simulink library "GOcontroll_Moduline_Target"  (R2018b)
settings: Solver=ode45  StartTime=0.0  StopTime=10.0  RelTol=1e-3  EnableMultiTasking=on
(part 1 of 3)
settings Model: Creator=HANcoder  LastModifiedBy=maud
settings Model: ModifiedHistory=|
  | la_obwlf -- Thu Sep 01 12:12:55 2016 -- Version 0.33
  | 
  | 
  | 
  | 
  | 
  | 
  | la_obwlf -- Thu Sep 01 09:23:34 2016 -- Version 0.33
  | changed the version in the Base Sample Time block
  | 
  | 
  | 
  | la_obwlf -- Tue Aug 30 15:48:17 2016 -- Version 0.33
settings DataIOCC: LimitDataPoints=on  SaveFormat=Array  SignalLoggingSaveFormat=ModelDataLogs
settings OptimizationCC: ExpressionDepthLimit=2147483647  LifeSpan=inf
settings DebuggingCC: UnderspecifiedInitializationDetection=Classic  MergeDetectMultiDrivingBlocksExec=none  SolverPrmCheckMsg=warning  FcnCallInpInsideContextMsg=warning  StateNameClashWarn=warning  SFUnexpectedBacktrackingDiag=warning  SFNoUnconditionalDefaultTransitionDiag=warning  SFExecutionAtInitializationDiag=none
settings HardwareCC: ProdBitPerPointer=32  ProdBitPerSizeT=32  ProdBitPerPtrDiffT=32  ProdLargestAtomicFloat=None  ProdIntDivRoundTo=Undefined  ProdEndianess=Unspecified  ProdWordSize=32  ProdHWDeviceType=32-bit Generic
settings ModelReferenceCC: PropagateSignalLabelsOutOfModel=off
settings SFSimCC: SimUseLocalCustomCode=off
settings RTWCC: RTWUseLocalCustomCode=off
settings CodeAppCC: StateflowObjectComments=on
settings GRTTargetCC: TargetLangStandard=C89/C90 (ANSI)  GeneratePreprocessorConditionals=Disable all  CombineOutputUpdateFcns=off  GRTInterface=on
settings ConfigComp: CovMetricSettings=dw  CovHtmlReporting=on  CovSaveCumulativeToWorkspaceVar=on  CovSaveSingleToWorkspaceVar=on  CovExternalEMLEnable=off  CovSFcnEnable=off

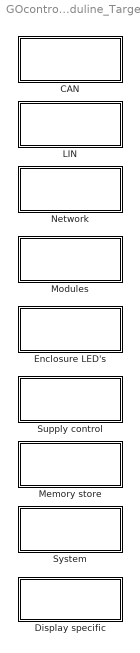
== system GOcontroll_Moduline_Target ==
  CAN : Subsystem
      mask Display: fprintf('CAN');
  Display specific : Subsystem
      mask Display: fprintf("Display specific");
  Enclosure LED's : Subsystem
      mask Display: fprintf('Enclosure LED');
  LIN : Subsystem
      mask Display: fprintf('LIN');
  Memory store : Subsystem
      mask Display: fprintf('Memory store');
  Modules : Subsystem
      mask Display: fprintf('Modules');
  Network : Subsystem
      mask Display: fprintf('Network');
  Supply control : Subsystem
      mask Display: fprintf('Supply Control');
  System : Subsystem
      mask Display: fprintf('System');

== system GOcontroll_Moduline_Target/CAN ==
  CAN 2.0B : Subsystem
      mask Display: fprintf('CAN 2.0B');

== system GOcontroll_Moduline_Target/Display specific ==
  Set display brightness : Subsystem  mask{tsamp=0}
      mask prompts: tsamp "Sample time:"
      mask help:
      | Set the brightness of a display (only works with the max25014 driver currently)
      | Keeps the original brightness untill the first non zero value is received
      mask init:
      | sfcn_set_brightness_display_mcb();
      mask Display:
      | fprintf("Set display brightness");
      | text(2, 6, ert_linux_target_version());

== system GOcontroll_Moduline_Target/Enclosure LED's ==
  Enclosure LED : Subsystem  Tag=HANcoder_GOcontroll_Moduline_IV  mask(Enclosure LED's){led=1, color=Red}
      mask help:
      | The Moduline controller is equipped with 4 RGB status LED's. To control them, simply configure the mask ( LED and color) and control them using uint8 values.
      |
      | Note: Moduline IV HW >= 3.02 has duty cycle controlled LED's. The intensity can be set from 0 (0%) to 255 (100%).
      |
      | LED: Select the LED that is needs to be controlled.
      |
      | Color: Select the color the LED needs to illuminate.
      mask init:
      | [colorInfoStr] = sfcn_gocontroll_status_led_mcb(led, color);
      mask TypeOptions led: 1 | 2 | 3 | 4
      mask TypeOptions color: Red | Green | Blue
      mask Display:
      | fprintf('Status LED %d\nColor: %s',led,colorInfoStr);
      | text(2, 6, ert_linux_target_version());

== system GOcontroll_Moduline_Target/LIN ==
  LIN Master : Subsystem  Tag=HANcoder_GOcontroll_Moduline_IV  mask(LIN Master){id=0x01, direction=Send data, dataLength=4, check=Classic (LIN 1.3), tsamp=-1}
      mask prompts: id "Identifier"; dataLength "Data Length"; check "Checksum"; tsamp "Sample time"
      mask help:
      | Function
      | ==========
      | This block implements the LIN master functionality for communication with LIN
      | slaves. The block complies with LIN 1.3 an LIN 2.0. When sending data to a slave
      | device, this block will add the data to the LIN bus. When retrieving data from slaves, The block will wait for incoming data over LIN.
      |
      | Parameters
      | ==========
      | Identifier:
      | Selects the identifier to communicate with
      |
      | Direction:
      | Request data from a slave device or send data to a slave device
      |
      | Datalength:
      | Defines the number of bytes that need to be send to- or requested from the slave
      |
      | Checksum:
      | Select Classic for checksum based on databytes only. Enhanced for databytes and
      | ID byte
      |
      | Sample time:
      | Defines the execution interval of the block.
      |
      | Input
      | ==========
      | Port 1..8               LIN Data bytes to be send to a slave
      |
      | Output
      | ==========
      | Port 1..8               LIN Data bytes that are received from the slave
      mask init:
      | sfcn_lin_master_mcb(id, direction, dataLength, check)
      mask TypeOptions id: 0x01 | 0x02 | 0x03 | 0x04 | 0x05 | 0x06 | 0x07 | 0x08 | 0x09 | 0x0A | 0x0B | 0x0C | 0x0D | 0x0E | 0x0F | 0x10 | 0x11 | 0x12 | 0x13 | 0x14 | 0x15 | 0x16 | 0x17 | 0x18 | 0x19 | 0x1A | 0x1B | 0x1C | 0x1D | 0x1E | 0x1F | 0x20 | 0x21 | 0x22 | 0x23 | 0x24 | 0x25 | 0x26 | 0x27 | 0x28 | 0x29 | 0x2A | 0x2B | 0x2C | 0x2D | 0x2E | 0x2F | 0x30 | 0x31 | 0x32 | 0x33 | 0x34 | 0x35 | 0x36 | 0x37 | 0x38 | 0x39 | 0x3A | 0x3B | 0x3C (diagnostic) | 0x3D (diagnostic) | 0x3E (reserved) | 0x3F (reserved)
      mask TypeOptions direction: Request data | Send data
      mask TypeOptions dataLength: 2 | 4 | 8
      mask TypeOptions check: Classic (LIN 1.3) | Enhanced (LIN 2.0)
      mask Display:
      | fprintf('Master LIN\nmessage\nID: 0x%x',id);
      | text(2, 6, ert_linux_target_version());

== system GOcontroll_Moduline_Target/Memory store ==
  Diagnostic to memory : Subsystem
      mask Display: fprintf('Diagnostic to memory');
  Variable to memory : Subsystem
      mask Display: fprintf('Variable to memory');

== system GOcontroll_Moduline_Target/Modules ==
  Bridge Module : Subsystem
      mask Display: fprintf('Bridge Module');
  Input Module : Subsystem
      mask Display: fprintf('Input Module');
  Output Module : Subsystem
      mask Display: fprintf('Output Module');

== system GOcontroll_Moduline_Target/Network ==
  MQTT : Subsystem
      mask Display: fprintf('MQTT');
  UDP : Subsystem
      mask Display: fprintf('UDP');

== system GOcontroll_Moduline_Target/Supply control ==
  Controller Active : Subsystem  Tag=HANcoder_GOcontroll_Moduline_IV  mask(Controller Active){tsamp=1}
      mask prompts: tsamp "Sample time"
      mask help:
      | The GOcontroll Moduline IV is able to keep itself alive. As long the K30 power is applied (connector C pin 5-7) and the input of the Controller Active function block is high, the controller will stay on even if the K15 pins (connector C pin 2,3 or 4) are low.
      | If the controller is switched off by software, a restart is only possible when the device is activated by one of the K15 pins of connector C.
      |
      | To detect an external shutdown (K15 pins goes low), simply drag in the K15 Voltage block. This block provides the input voltage from the K15 pins
      mask init:
      | sfcn_gocontroll_controller_active_mcb();
      mask Display:
      | fprintf('Controller Active');
      | text(2, 6, ert_linux_target_version());
  K15 Voltage : Subsystem  Tag=HANcoder_GOcontroll_Moduline_IV  mask(Contact Voltage){tsamp=1, k15pin=K15-1 (Connector C pin 2)}
      mask prompts: tsamp "Sample time"; k15pin "K15 input pin"
      mask help: The K15 voltage provides the K15 voltage in mV that is applied on connector C pin 2,3 or 4. A positive voltage on one of these pins will start-up the controller. These function blocks can be used to read out which K15 input pin triggered the startup.
      mask init:
      | sfcn_gocontroll_k15_voltage_mcb(k15pin);
      mask TypeOptions k15pin: K15-1 (Connector C pin 2) | K15-2 (Connector C pin 3) | K15-3 (Connector C pin 4)
      mask Display:
      | fprintf('K15 Voltage\nConnector C pin %d',k15pin+1);
      | text(2, 6, ert_linux_target_version());
  K30 Voltage : Subsystem  Tag=HANcoder_GOcontroll_Moduline_IV  mask(Supply voltage){tsamp=1}
      mask prompts: tsamp "Sample time"
      mask help: The K30 voltage provides the power supply in mV that is applied on connector C pin 5-7
      mask init:
      | sfcn_gocontroll_k30_voltage_mcb();
      mask Display:
      | fprintf('K30 Voltage\nConnector C pin 5-7');
      | text(2, 6, ert_linux_target_version());

== system GOcontroll_Moduline_Target/System ==
  Build Settings : Subsystem  Tag=HANcoder_GOcontroll_Moduline_IV  mask{AutoASAP2add=on, AutoFlash=off}
      mask prompts: AutoASAP2add "Add signals and parameters automatically"; AutoFlash "Automatic flash after build"
      mask TypeOptions AutoASAP2add: on | off
      mask TypeOptions AutoFlash: off | USB | CAN | Ethernet
      mask DialogControl ParameterTabVar0 Prompt: Auto Add
      mask DialogControl Control3 Prompt: With this option the undefined parameters and signals will automatically be added to the workspace for use with HANtune. You will be prompted for the parameter values.
      mask DialogControl ParameterTabVar01 Prompt: Auto Flash
      mask DialogControl Control2 Prompt: With this option you can choose to automatically start MicroBoot after the build is complete. MicroBoot will start flashing using the selected interface.
      mask Display:
      | fprintf('Build settings\nAuto Add: %s\nAuto Flash: %s',AutoASAP2add, AutoFlash);
      | text(2, 6, ert_linux_target_version());
  CPU : Subsystem  Tag=HANcoder_GOcontroll_Moduline_IV  mask(Get CPU temperature){tsamp=1}
      mask prompts: tsamp "Sample time"
      mask help: Function block to retrieve the CPU temperature from the i.MX core
      mask init:
      | sfcn_gocontroll_cpu_temperature_mcb();
      mask Display:
      | fprintf('Get CPU temperature');
      | text(2, 6, ert_linux_target_version());
  Execute Shell Command : M-S-Function  FunctionName=sfcn_exec_shell  Parameters=tsamp,command  mask{command=command, tsamp=1}
      mask prompts: tsamp "Sample time:"
      mask help: Execute a Linux Shell command when the input is true
      mask init:
      | sfcn_exec_shell_mcb(command);
      mask Help: Accepts a Boolean input, potentially use a triggered subsystem to call the function only once on a state change.
      mask Display:
      | fprintf("Execute command:\n%s",command);
      | text(2, 6, ert_linux_target_version());
  License Key : Subsystem  Tag=HANcoder_GOcontroll_Moduline_IV  mask(Check software license key){tsamp=1, key=key, iv=initVec, license=/path/to/file, check_file=/path/to/file}
      mask prompts: tsamp "Sample time"; key "Encryption key"; iv "Initialisation vector"; license "License file"; check_file "Check file"
      mask help: Function block to check the controller for a license key upon executing the software.
      mask init:
      | sfcn_license_key_mcb(key,iv,license,check_file);
      mask Help:
      | example lines are literal,  {}s need to be present in the text fields.
      | 
      | Encryption key:
      | 
      | An array of 16, 24 or 32 bytes, for example:
      | {0x01, 0x23, 0x45, 0x67, 0x89, 0xAB, 0xCD, 0xEF, 0x01, 0x23, 0x45, 0x67, 0x89, 0xAB, 0xCD, 0xEF}
      | 
      | bytes can be written in any form accepted by the c compiler: 0x00/0 to 0xFf/255.
      | 
      | Inititialisation vector:
      | 
      | A string of characters (max 16 bytes) example:
      | 123kdgh34ndfg84
      | 
      | 
      | License file:
      | 
      | A string containing the path to the license file, example:
      | /etc/simulink/license
      | 
      | 
      | Check file:
      | 
      | A string containing the path to the license file, example:
      | /etc/simulink/check_file
      | 
      | 
      | Method of operation:
      | This block uses the <a href="https://github.com/jhjin/OpenAES">OpenAES library</a>. It also has a tool that can be used to generate an encryption key and to encrypt a file with said key.
      | 
      | This block will attempt to decrypt the "license file" with the given key and initialisation vector, it will then be compared to the "check file". If these match the program is allowed to continue.
      | 
      | To make this work effectively it is essential to encrypt a file that is unique for the system and can't be easily edited. for example "/sys/class/net/eth0/address".
      | 
      | An important note with using this block is that the bytes of the key are swapped and so need to be entered slightly differently in this block, for example:
      | key: byte 1 byte 2 byte 3 byte 4 byte 5 byte 6 ...
      | block: {byte 2, byte 1, byte 4, byte 3, byte 6, byte 5, ...}
      | 
      | If the model terminates with the error:
      | Error: Failed to decrypt2. return code: ##
      | 
      | It means the license key is faulty and needs to be checked in the block.
      | it might be that your system does display the key in the right order for the block, so if this error happens first double check, then try swapping them to the regular order.
      mask Display:
      | fprintf('Check software license');
      | text(2, 6, ert_linux_target_version());

== system GOcontroll_Moduline_Target/CAN/CAN 2.0B ==
  CAN receive1 : Subsystem  Tag=HANcoder_GOcontroll_Moduline_IV  mask(CAN receive){canBus=CAN1 - Connector C pin 14 (L) and pin 15 (H), outputNumber=1, dataType=uint8, byteOrder=on, tsamp=-1}
      mask prompts: canBus "CAN channel"; outputNumber "Output ports"; dataType "Output datatype"; byteOrder "Byte order: Checked = MSB first, unchecked = LSB first."; tsamp "Sample time"
      mask help:
      | Function
      | ==========
      | Receive the newest message from the specified CAN channel.
      |
      | Parameters
      | ==========
      | CAN channel:             The CAN channel to send the message on.
      | Output ports:             The amount of output ports
      | Output datatype:       The datatype of the output ports
      | Byte order:                 Select MSB or LSB first
      | Sample time:              -1 or divisible by base sample time [seconds]
      |
      | Input
      | ==========
      | Port 1:                       CAN ID(uint32) in hexadecimal ie: hex2dec('0a')
      |
      | Output
      | ==========
      | Port 1:                       Checks for new message(int8)
      | Port 2..9                     Message data
      mask init:
      | sfcn_can_receive_mcb(canBus, outputNumber, dataType, byteOrder)
      | 
      | % Get current number of outputs & inputs ('gcb' is a system defined var that points
      | % to the tree structure of the current block)
      | currentOutputNumber = 0;
      | for i = 1:9
      |     if (getSimulinkBlockHandle([gcb, '/Out', num2str(i)]) ~= -1)
      |         currentOutputNumber = currentOutputNumber + 1;
      |     end
      | end
      | % Now we update the number of outputs to match the given amount
      | % If we have to many outputs (-1 for the 'new data' port):
      | if currentOutputNumber - 1 > outputNumber
      |     % Loop trough all outputs that are to much
      |     for counterRemove = outputNumber+2:currentOutputNumber
      |         if (getSimulinkBlockHandle([gcb, '/Out', num2str(counterRemove)]) ~= -1)
      |             % Get the position of the output block
      |             thisPosition = get_param ([gcb, '/Out', num2str(counterRemove)], 'Position');
      |             % Remove the output block
      |             delete_block ([gcb, '/Out', num2str(counterRemove)])
      |             % Add a terminator block
      |             add_block ('built-in/Terminator', [gcb, '/Term', num2str(counterRemove)])
      |             % Align the new terminator block to be placed at the position of the
      |             % removed output
      |             set_param ([gcb, '/Term', num2str(counterRemove)], 'Position', thisPosition)
      |         end
      |     end
      | % Or if we have to few inputs (-1 for the 'new data' port):
      | elseif outputNumber > currentOutputNumber - 1
      |     % Loop trough all terminators that needs to be outputs
      |     for counterAdd = currentOutputNumber+1:outputNumber+1
      |         if (getSimulinkBlockHandle([gcb, '/Term', num2str(counterAdd)]) ~= -1)
      |             % Get the position of the terminator block
      |             thisPosition = get_param ([gcb, '/Term', num2str(counterAdd)], 'Position');
      |             % Remove the terminator block
      |             delete_block ([gcb, '/Term', num2str(counterAdd)])
      |             % Add a output block
      |             add_block ('built-in/Outport', [gcb, '/Out', num2str(counterAdd)])
      |             % Align the new output block to be placed at the position of the
      |             % removed terminator
      |             set_param ([gcb, '/Out', num2str(counterAdd)], 'Position', thisPosition)
      |         end
      |     end
      | end
      mask Help: web('sfcn_can_receive.html');
      mask TypeOptions canBus: CAN1 - Connector C pin 14 (L) and pin 15 (H) | CAN2 - Connector C pin 20 (L) and pin 21 (H) | CAN3 - Connector C pin 19 (L) and pin 18 (H) | CAN4 - Connector C pin 13 (L) and pin 12 (H)
      mask TypeOptions dataType: int8 | uint8 | int16 | uint16 | int32 | uint32 | boolean
      mask Display:
      | fprintf('Receive on\nCAN %x', canBus);
      | port_label('output', 1, 'new')
      | port_label('input', 1, 'ID');
      | text(2, 6, ert_linux_target_version());
  CAN send1 : Subsystem  Tag=HANcoder_GOcontroll_Moduline_IV  mask(CAN send){canBus=CAN1 - Connector C pin 14 (L) and pin 15 (H), frameType=Standard (11 bit), inputNumber=2, dataType=uint8, byteOrder=on, RTR=off, tsamp=-1}
      mask prompts: canBus "CAN channel"; frameType "Identifier type"; inputNumber "Input ports"; dataType "Input datatype"; byteOrder "Byte order: Checked = MSB first, unchecked = LSB first."; RTR "Remote Transmission Request"; tsamp "Sample time"
      mask help:
      | Function
      | ==========
      | Send a message on the CAN channel.
      |
      | Parameters
      | ==========
      | CAN channel:           The CAN channel to send the message on.
      | Identifier type:         normal or extended ID's
      | Input ports:              The amount of input ports
      | Input datatype:        The datatype of the input ports
      | Byte order:               Select MSB or LSB first
      | Sample time:            -1 or divisible by base sample time [seconds]
      |
      | Input
      | ==========
      | Port 1:                   CAN ID(uint32) in hexadecimal ie: hex2dec('0a')
      | Port 2..9                CAN message data
      mask init:
      | sfcn_can_send_mcb(canBus, frameType, inputNumber, dataType, byteOrder, RTR)
      | 
      | % Get current number of outputs & inputs ('gcb' is a system defined var that points
      | % to the tree structure of the current block)
      | currentInputNumber = 0;
      | for i = 1:9
      |     if (getSimulinkBlockHandle([gcb, '/In', num2str(i)]) ~= -1)
      |         currentInputNumber = currentInputNumber + 1;
      |     end
      | end
      | % Now we update the number of outputs to match the given amount
      | % If we have to many inputs (-1 for the 'new data' port):
      | if inputNumber < currentInputNumber - 1
      |     % Loop trough all outputs that are to much
      |     for counterRemove = inputNumber+2:currentInputNumber
      |         if (getSimulinkBlockHandle([gcb, '/In', num2str(counterRemove)]) ~= -1)
      |             % Get the position of the output block
      |             thisPosition = get_param ([gcb, '/In', num2str(counterRemove)], 'Position');
      |             % Remove the output block
      |             delete_block ([gcb, '/In', num2str(counterRemove)])
      |             % Add a terminator block
      |             add_block ('built-in/Ground', [gcb, '/Gnd', num2str(counterRemove)])
      |             % Align the new terminator block to be placed at the position of the
      |             % removed output
      |             set_param ([gcb, '/Gnd', num2str(counterRemove)], 'Position', thisPosition)
      |         end
      |     end
      | % Or if we have to few inputs (-1 for the 'new data' port):
      | elseif inputNumber > currentInputNumber - 1
      |     % Loop trough all terminators that needs to be outputs
      |     for counterAdd = currentInputNumber+1:inputNumber+1
      |         if (getSimulinkBlockHandle([gcb, '/Gnd', num2str(counterAdd)]) ~= -1)
      |             % Get the position of the terminator block
      |             thisPosition = get_param ([gcb, '/Gnd', num2str(counterAdd)], 'Position');
      |             % Remove the terminator block
      |             delete_block ([gcb, '/Gnd', num2str(counterAdd)])
      |             % Add a output block
      |             add_block ('built-in/Inport', [gcb, '/In', num2str(counterAdd)])
      |             % Align the new output block to be placed at the position of the
      |             % removed terminator
      |             set_param ([gcb, '/In', num2str(counterAdd)], 'Position', thisPosition)
      |         end
      |     end
      | end
      mask Help: web('sfcn_can_send.html');
      mask TypeOptions canBus: CAN1 - Connector C pin 14 (L) and pin 15 (H) | CAN2 - Connector C pin 20 (L) and pin 21 (H) | CAN3 - Connector C pin 19 (L) and pin 18 (H) | CAN4 - Connector C pin 13 (L) and pin 12 (H)
      mask TypeOptions frameType: Standard (11 bit) | Extended (29 bit)
      mask TypeOptions dataType: int8 | uint8 | int16 | uint16 | int32 | uint32 | boolean
      mask Display:
      | fprintf('Send on\nCAN%x', canBus);
      | port_label('input', 1, 'ID');
      | if RTR
      |     fprintf('\n\n\n\nRTR');
      | end
      | text(2, 6, ert_linux_target_version());

== system GOcontroll_Moduline_Target/Display specific/Set display brightness ==
  brightness : Inport
  Level-2 MATLAB S-Function : M-S-Function  FunctionName=sfcn_set_brightness_display  Parameters=tsamp
  wires:
  brightness/1 -> Level-2 MATLAB S-Function/1

== system GOcontroll_Moduline_Target/Enclosure LED's/Enclosure LED ==
  In1 : Inport
  S-Function : M-S-Function  FunctionName=sfcn_gocontroll_status_led  Parameters=led, color
  wires:
  In1/1 -> S-Function/1

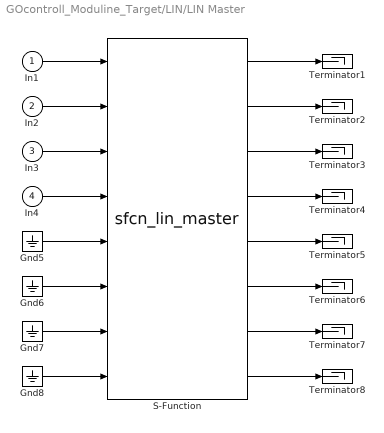
== system GOcontroll_Moduline_Target/LIN/LIN Master ==
  In1 : Inport
  In2 : Inport  Port=2
  In3 : Inport  Port=3
  In4 : Inport  Port=4
  Gnd{5..8} (4 alike) : Ground
  S-Function : M-S-Function  FunctionName=sfcn_lin_master  Parameters=tsamp, id, direction, dataLength, check
  Terminator{1..8} (8 alike) : Terminator
  wires:
  Gnd8/1 -> S-Function/8
  Gnd7/1 -> S-Function/7
  Gnd6/1 -> S-Function/6
  Gnd5/1 -> S-Function/5
  In4/1 -> S-Function/4
  In3/1 -> S-Function/3
  In2/1 -> S-Function/2
  In1/1 -> S-Function/1
  S-Function/1 -> Terminator1/1
  S-Function/2 -> Terminator2/1
  S-Function/3 -> Terminator3/1
  S-Function/4 -> Terminator4/1
  S-Function/5 -> Terminator5/1
  S-Function/6 -> Terminator6/1
  S-Function/7 -> Terminator7/1
  S-Function/8 -> Terminator8/1

== system GOcontroll_Moduline_Target/Memory store/Diagnostic to memory ==
  Delete all codes for one group : Subsystem  Tag=HANcoder_GOcontroll_Moduline_IV  mask(Delete diagnostic codes from memory){tsamp=0.5, diagType=Warning}
      mask prompts: tsamp "Sample time"; diagType "Diagnostic code type:"
      mask help:
      | This function block deletes stored codes under the specified diagnostic code type.
      |
      | Sample time:
      | -1 for inherited since this block is a triggered system
      |
      | Diagnostic code type:
      | The type defines the severity of the diagnostic code categorie that is deleted.
      mask init:
      | diagCodeDescription = sfcn_memory_diagnostic_delete_code_mcb(diagType);
      mask TypeOptions diagType: Warning | Warning with action | Error | Error with action | Fatal Error
      mask Display:
      | fprintf('Delete all codes for:\n%s',diagCodeDescription);
      | text(2, 6, ert_linux_target_version());
  Number of stored diagnostic codes : Subsystem  Tag=HANcoder_GOcontroll_Moduline_IV  mask(Read number of stored codes){tsamp=0.5, diagType=Warning}
      mask prompts: tsamp "Sample time"; diagType "Diagnostic code type:"
      mask help:
      | This function block reads the number of stored codes under the specified diagnostic code type.
      |
      | Sample time:
      | Execution period for the function block.
      |
      | Diagnostic code type:
      | The type defines the severity of the diagnostic code categorie that is read.
      mask init:
      | diagCodeDescription = sfcn_memory_diagnostic_nrcodes_read_mcb(diagType);
      mask TypeOptions diagType: Warning | Warning with action | Error | Error with action | Fatal Error
      mask Display:
      | fprintf('Get number of codes for:\n%s',diagCodeDescription);
      | text(2, 6, ert_linux_target_version());
  Read diagnostic code : Subsystem  Tag=HANcoder_GOcontroll_Moduline_IV  mask(Read a diagnostic code from memory){tsamp=0.5}
      mask prompts: tsamp "Sample time"
      mask help:
      | This function block reads a stored diagnostic code from a specified diagnostic type. The code that is read from memory is specified by the index numper on input port 2. The stored code goes out of the functionblock as a uint32 value.
      |
      | Sample time:
      | Execution period for the function block.
      mask init:
      | sfcn_memory_diagnostic_read_code_mcb();
      mask Display:
      | fprintf('Read diagnostic code\nfrom index');
      | port_label('input', 1, 'Diagnostic type');
      | port_label('input', 2, 'Index');
      | port_label('output', 1, 'Code');
      | text(2, 6, ert_linux_target_version());
  Store diagnostic code : Subsystem  Tag=HANcoder_GOcontroll_Moduline_IV  mask(Store diagnostic code to memory){tsamp=-1, diagType=Warning}
      mask prompts: tsamp "Sample time:"; diagType "Diagnosic code type:"
      mask help:
      | This function block stores a diagnostic code to memory including maximal 10 freezed frame parameters. Once a rising edge on the trigger input is detected. The diagnostic code on input 1 and the freezed frame parameters on input 2 to 11 are stored to memory.
      |
      | Sample time:
      | -1 here for inherited since this function block is a triggered system.
      |
      | Diagnostic code type:
      | The type defines the severity of the diagnostic code.
      mask init:
      | diagCodeDescription = sfcn_memory_diagnostic_write_code_mcb(diagType);
      mask TypeOptions diagType: Warning | Warning with action | Error | Error with action | Fatal Error
      mask Display:
      | fprintf('Store diagnostic code\nin memory\nType: %s', diagCodeDescription);
      | port_label('input', 1, 'Diagnostic code');
      | text(2, 6, ert_linux_target_version());
  Store diagnostic code with freeze frame : Subsystem  Tag=HANcoder_GOcontroll_Moduline_IV  mask(Store diagnostic code to memory with freezed frame){tsamp=-1, diagType=Warning, FreezeParam1=Param1, FreezeParam2=Param2, FreezeParam3=Param3, FreezeParam4=Param4, FreezeParam5=Param5, FreezeParam6=Param6, FreezeParam7=Param7, FreezeParam8=Param8, FreezeParam9=Param9, FreezeParam10=Param10}
      mask prompts: tsamp "Sample time:"; diagType "Diagnosic code type:"; FreezeParam1 "Freezed frame parameter 1:"; FreezeParam2 "Freezed frame parameter 2:"; FreezeParam3 "Freezed frame parameter 3:"; FreezeParam4 "Freezed frame parameter 4:"; FreezeParam5 "Freezed frame parameter 5:"; FreezeParam6 "Freezed frame parameter 6:"; FreezeParam7 "Freezed frame parameter 7:"; FreezeParam8 "Freezed frame parameter 8:"; FreezeParam9 "Freezed frame parameter 9:"; FreezeParam10 "Freezed frame parameter 10:"
      mask help:
      | This function block stores a diagnostic code to memory including maximal 10 freezed frame parameters. Once a rising edge on the trigger input is detected. The diagnostic code on input 1 and the freezed frame parameters on input 2 to 11 are stored to memory.
      |
      | Sample time:
      | -1 here for inherited since this function block is a triggered system.
      |
      | Diagnostic code type:
      | The type defines the severity of the diagnostic code.
      |
      | Freezed frame parameter x:
      | This describes the signal on the coresponding input. This description is stored along with the signal in the freezed frame.
      mask init:
      | diagCodeDescription = sfcn_memory_diagnostic_write_freeze_mcb(diagType,FreezeParam1,FreezeParam2,FreezeParam3,FreezeParam4,...
      | 								FreezeParam5,FreezeParam6,FreezeParam7,FreezeParam8,FreezeParam9,...
      |                                 FreezeParam10);
      mask TypeOptions diagType: Warning | Warning with action | Error | Error with action | Fatal Error
      mask Display:
      | fprintf('Store diagnostic code\nin memory with freezed frame\nType: %s', diagCodeDescription);
      | port_label('input', 1, 'Diagnostic code');
      | port_label('input', 2, FreezeParam1);
      | port_label('input', 3, FreezeParam2);
      | port_label('input', 4, FreezeParam3);
      | port_label('input', 5, FreezeParam4);
      | port_label('input', 6, FreezeParam5);
      | port_label('input', 7, FreezeParam6);
      | port_label('input', 8, FreezeParam7);
      | port_label('input', 9, FreezeParam8);
      | port_label('input', 10, FreezeParam9);
      | port_label('input', 11, FreezeParam10);
      | text(2, 6, ert_linux_target_version());

== system GOcontroll_Moduline_Target/Memory store/Variable to memory ==
  Memory read : Subsystem  Tag=HANcoder_GOcontroll_Moduline_IV  mask(Read value from memory){memRead=Read once during startup, memType=Non-persistant Memory (RAM), tsamp=1, key=key1, init=0}
      mask prompts: memRead "Memory read"; memType "Memory type"; tsamp "Sample time"; key "Key 1:"; init "Initialization value:"
      mask help: This function block reads a value from memory by the specified key. To store a value to memory, use the store to memory function block.
      mask init:
      | sfcn_memory_emulation_read_mcb(memRead,memType,key,init);
      mask TypeOptions memRead: Read once during startup | Read periodic based on sample time
      mask TypeOptions memType: Persistant Memory (eMMC) | Non-persistant Memory (RAM)
      mask Display:
      | fprintf('Read from memory\nKey: %s',key);
      | text(2, 6, ert_linux_target_version());
  Memory write : Subsystem  Tag=HANcoder_GOcontroll_Moduline_IV  mask(Store data to memory){memType=Non-persistant Memory (RAM), tsamp=1, key=key1}
      mask prompts: memType "Memory type"; tsamp "Sample time:"; key "Key 1:"
      mask help: This function block stores a value to the memory with a specified key. To get the stored value from memory, use the read from memory function block and retrieve the value by key
      mask init:
      | sfcn_memory_emulation_write_mcb(key, memType);
      mask TypeOptions memType: Persistant Memory (eMMC) | Non-persistant Memory (RAM)
      mask Display:
      | fprintf('Store in memory\nKey: %s',key);
      | text(2, 6, ert_linux_target_version());

== system GOcontroll_Moduline_Target/Modules/Bridge Module ==
  Bridge Module : Subsystem  Tag=HANcoder_GOcontroll_Moduline_IV  mask(Bridge Module){tsamp=-1, ContrType=GOcontroll Moduline IV, moduleSlot=Module slot 1, C1func=Disable (output disabled), C1freq=200 Hz, C2func=Disable (output disabled), C2freq=200 Hz}
      mask prompts: tsamp "Sample time"; ContrType "Controller Type"; moduleSlot "Module Slot"; C1func "Function select"; C1freq "Frequency"; C2func "Function select"; C2freq "Frequency"
      mask help:
      | With this function block, you can configure each output of the bridge module (202001xx). During initialization of the controller, the corresponding outputs of the module are set according the settings. During runtime, the value pushed into the block will control the outputs.
      |
      | Module slot:
      | Sets the location of the module slot where the module is physically
      | plugged into.
      |
      | Channel tabs:
      | Each ouput has its own configuration tab.
      |
      | Function select:
      | Select the desired output configuration.
      |
      | Frequency:
      | In case a duty Cycle is used, select the frequency.
      mask init:
      | [moduleSlotInfoStr, connectorId, pin1Id, pin2Id] = sfcn_gocontroll_bridge_module_mcb(moduleSlot,ContrType,C1func,C1freq,C2func,C2freq);
      | [version] = ert_linux_target_version();
      settings: MoveFcn=%%drawLogos
      mask TypeOptions ContrType: GOcontroll Moduline IV | GOcontroll Moduline Mini | GOcontroll Moduline Display
      mask Callback ContrType:
      | msk = Simulink.Mask.get(gcb);
      | p = msk.Parameters;
      | 
      | func = get_param(gcb,'ContrType');
      | 
      | if(func == "GOcontroll Moduline IV")
      | p(3).TypeOptions = {'Moduleslot 1','Moduleslot 2','Moduleslot 3','Moduleslot 4',...
      |                     'Moduleslot 5','Moduleslot 6','Moduleslot 7','Moduleslot 8'};
      | 
      | elseif (func == "GOcontroll Moduline Mini")
      |  p(3).TypeOptions = {'Moduleslot 1','Moduleslot 2','Moduleslot 3','Moduleslot 4'};
      | 
      | elseif (func == "GOcontroll Moduline Screen")
      |  p(3).TypeOptions = {'Moduleslot 1','Moduleslot 2'};
      | 
      | end
      mask TypeOptions moduleSlot: Module slot 1 | Module slot 2 | Module slot 3 | Module slot 4 | Module slot 5 | Module slot 6 | Module slot 7 | Module slot 8
      mask TypeOptions C1func: Disable (output disabled) | Half Bridge dutycycle controlled 0% - 100% duty cycle ( 0 - 1000) | Low side switch  dutycycle controlled 0% - 100% duty cycle (0 - 1000) | High side switch  dutycycle controlled 0% - 100% duty cycle (0 - 1000) | Low side switch On - Off (1-0) | High side switch On - Off (1-0)
      mask TypeOptions C1freq: 100 Hz | 200 Hz | 500 Hz | 1 kHz | 2 kHz | 5 kHz | 10 kHz
      mask TypeOptions C2func: Disable (output disabled) | Half Bridge dutycycle controlled 0% - 100% duty cycle ( 0 - 1000) | Low side switch  dutycycle controlled 0% - 100% duty cycle (0 - 1000) | High side switch  dutycycle controlled 0% - 100% duty cycle (0 - 1000) | Low side switch On - Off (1-0) | High side switch On - Off (1-0)
      mask TypeOptions C2freq: 100 Hz | 200 Hz | 500 Hz | 1 kHz | 2 kHz | 5 kHz | 10 kHz
      mask DialogControl Container4 Prompt: Output 1
      mask DialogControl Container5 Prompt: Output 2
      mask Display:
      | fprintf('Bridge Module\n%s\n\n Controller Connector: %s', moduleSlotInfoStr,connectorId);
      | port_label('input', 1, pin1Id);
      | port_label('input', 2, pin2Id);
      | text(2, 6, ert_linux_target_version());
  Bridge Module Monitor : Subsystem  Tag=HANcoder_GOcontroll_Moduline_IV  mask(Bridge Module Monitor){tsamp=-1, ContrType=GOcontroll Moduline IV, moduleSlot=Module slot 1}
      mask prompts: tsamp "Sample time"; ContrType "Controller Type"; moduleSlot "Module Slot"
      mask help:
      | With this function block, you can read parameters from the specified bridge module (202001xx). The block will provide some information about the module such as:
      |
      | Module temperature:
      | The temperature in degrees from the output module.
      |
      | Module ground shift
      | In case the ground connection of the module is poor, the power ground is shifted. The value gives the ground difference in mV and schould be beneath 50 mV
      |
      | Channel current
      | Current related output for each output channel
      mask init:
      | [moduleSlotInfoStr, connectorId, pin1Id, pin2Id] = sfcn_gocontroll_bridge_module_monitor_mcb(moduleSlot,ContrType);
      settings: MoveFcn=%%drawLogos
      mask TypeOptions ContrType: GOcontroll Moduline IV | GOcontroll Moduline Mini | GOcontroll Moduline Display
      mask Callback ContrType:
      | msk = Simulink.Mask.get(gcb);
      | p = msk.Parameters;
      | 
      | func = get_param(gcb,'ContrType');
      | 
      | if(func == "GOcontroll Moduline IV")
      | p(3).TypeOptions = {'Moduleslot 1','Moduleslot 2','Moduleslot 3','Moduleslot 4',...
      |                     'Moduleslot 5','Moduleslot 6','Moduleslot 7','Moduleslot 8'};
      | 
      | elseif (func == "GOcontroll Moduline Mini")
      |  p(3).TypeOptions = {'Moduleslot 1','Moduleslot 2','Moduleslot 3','Moduleslot 4'};
      | 
      | elseif (func == "GOcontroll Moduline Screen")
      |  p(3).TypeOptions = {'Moduleslot 1','Moduleslot 2'};
      | 
      | end
      mask TypeOptions moduleSlot: Module slot 1 | Module slot 2 | Module slot 3 | Module slot 4 | Module slot 5 | Module slot 6 | Module slot 7 | Module slot 8
      mask Display:
      | fprintf('Bridge Module Monitor\n%s\n\n Controller Connector: %s', moduleSlotInfoStr,connectorId);
      | port_label('output', 1, 'Temperature');
      | port_label('output', 2, 'Groundshift');
      | port_label('output', 3, pin1Id);
      | port_label('output', 4, pin2Id);
